simulink model "DR18E_Testpult"  (R2017a)
settings: Solver=ode1  StartTime=0.0  StopTime=Inf  FixedStep=0.001  RelTol=1e-3
PostLoadFcn:
  | , if any(exist('dsrtsu_mdlpostloadfcn', 'file') == [2, 3, 6]), try dsrtsu_mdlpostloadfcn('Execute', bdroot); catch fprintf('Error in PostLoadFcn (dsrtsu_mdlpostloadfcn) for model "%s":\n %s\n', bdroot, lasterr); end, end,
model workspace: external: MAT-File C:\Users\DeltaRacing\Documents\dSPACE\MABX_DR18E\Model\DR18E_MABX_Parameter.mat (data not in the file)
values from neighbouring files (symbols this model uses):
  am = 1/Ts    (= 1)    [DR18E_MABX_Parameter.m]
  bm = K/Ts    (= 0.05)    [DR18E_MABX_Parameter.m]
  cf = 41350    [DR18E_MABX_Parameter.m]
  cr = 41350    [DR18E_MABX_Parameter.m]
  Derating_HV_Battery_Kapa = 1    [DR18E_MABX_Parameter.m]
  Derating_Start_km = 16    [DR18E_MABX_Parameter.m]
  Drive_Mode = 0    [DR18E_MABX_Parameter.m]
  g = 1    [DR18E_MABX_Parameter.m]
  Gas_Modus = 2    [DR18E_MABX_Parameter.m]
  HV_Power_max = 80    [DR18E_MABX_Parameter.m]
  i_Getriebe = 3.3    [DR18E_MABX_Parameter.m]
  i_Lenkgetriebe = 4.32    [DR18E_MABX_Parameter.m]
  K_SET = 1    [DR18E_MABX_Parameter.m]
  Kapazitaet_HV_Battery_kWh = 6.6    [DR18E_MABX_Parameter.m]
  KW_T_Soll = 37    [DR18E_MABX_Parameter.m]
  lf = 1.2    [DR18E_MABX_Parameter.m]
  lr = 1.15    [DR18E_MABX_Parameter.m]
  m = mdriver + mvehicle    (= 310)    [DR18E_MABX_Parameter.m]
  M_max = 150    [DR18E_MABX_Parameter.m]
  Power_Limit_onoff = 0    [DR18E_MABX_Parameter.m]
  Reifenradius = 0.2351    [DR18E_MABX_Parameter.m]
  Strecke_Endu_km = 22    [DR18E_MABX_Parameter.m]
  TC_Decr_Gas = 0.00005    (= 5e-05)    [DR18E_MABX_Parameter.m]
  TC_Derivative = 0.4    [DR18E_MABX_Parameter.m]
  TC_Incr_Gas = 0.005    [DR18E_MABX_Parameter.m]
  TC_On = 0    [DR18E_MABX_Parameter.m]
  TC_Relay_Off = 0.065    [DR18E_MABX_Parameter.m]
  TC_Relay_On = 0.07    [DR18E_MABX_Parameter.m]
  TV_Mode = 2    [DR18E_MABX_Parameter.m]
  TV_On = 0    [DR18E_MABX_Parameter.m]
  TV_Override = 1    [DR18E_MABX_Parameter.m]
  y = 0.8    [DR18E_MABX_Parameter.m]
undefined symbols (not defined in the file or in its folder): D, DiscIntNeverNeededParam, I, K_OL, P
libraries: simulink x288, rtican x100, rtiusbflightreclib x40, rti1401lib_dio_type3 x10, simulink_extras x10, rti1401lib_adc_type4 x8, rti1401lib_II_base x7
(part 25 of 27)

== system DR18E_Testpult/Verarbeitung/Bremse/PlausibilityCheck/PT1 Discrete1 ==
  u : Inport
  K : Inport  Port=2
  T : Inport  Port=3
  Memory : Memory
  Product : Product
  Product1 : Product
  Subsystem : Subsystem
  Sum : Sum  Inputs=|+-
  Sum1 : Sum  Inputs=|++
  y : Outport
  wires:
  T/1 -> Subsystem/1(T)
  Product/1 -> Sum/1
  Sum1/1 -> Memory/1, y/1
  Memory/1 -> Sum/2, Sum1/2
  Product1/1 -> Sum1/1
  Sum/1 -> Product1/2
  u/1 -> Product/2
  Subsystem/1(T*) -> Product1/1
  K/1 -> Product/1

== system DR18E_Testpult/Verarbeitung/DR18E Torque Control/Derating/Derating_Strategie_Reichweite ==
  note: Eingänge Timeout Drehzahlsensor
      | HV Strom
  In1 : Inport
  In2 : Inport  Port=2
  Add : Sum  Inputs=+-
  Add1 : Sum  Inputs=-+
  Add2 : Sum  Inputs=-+
  Compare To Constant : simulink/Logic and Bit Operations/Compare To Constant  relop===  const=3.0  OutDataTypeStr=boolean
  Constant : Constant  Value=Kapazitaet_HV_Battery_kWh
  Constant1 : Constant  Value=Strecke_Endu_km
  Constant2 : Constant  Value=Drive_Mode
  Constant3 : Constant  Value=Derating_HV_Battery_Kapa
  Constant4 : Constant  Value=Derating_Start_km
  Derating_Battery_active : Switch  Criteria=u2 > Threshold
  Divide : Product  Inputs=*/
  Divide1 : Product  Inputs=*/
  Logical Operator : Logic  Inputs=4  AllPortsSameDT=off  OutDataTypeStr=boolean
  Map_Reichweite_Derating_Rev1 : Lookup_n-D  NumberOfTableDimensions=1  BreakpointsForDimension1=[0;1;2;3;4;5;6;7;8;9;10]  Table=[1;0.9;0.8;0.8;0.8;0.8;0.8;0.7;0.7;0.7;0.7]  InternalRulePriority=Speed  RndMeth=Simplest  InputSameDT=on
  Relational Operator : RelationalOperator  OutDataTypeStr=boolean  RndMeth=Simplest
  Safety1 : Constant  Value=0
  Safety_Derateing : Constant
  Saturation : Saturate  UpperLimit=10  LowerLimit=0
  Verbrauch_Wh/km : Subsystem
  kWh->Wh : Gain  Gain=1000
  m->km : Gain  Gain=1/1000
  deltaStrecke_km : Outport
  Derating_RW_aktivate_bin : Outport  Port=2
  wires:
  Add1/1 -> Add2/2  "Reststrecke_km"
  Add/1 -> Divide1/1  "verbleibendeEnergie_Wh"
  kWh->Wh/1 -> Add/1
  Divide1/1 -> Add2/1  "Restreichweite_km"
  In1/1 -> Divide/1, Add/2
  m->km/1 -> Relational Operator/1, Add1/1, Divide/2
  Constant1/1 -> Add1/2
  Constant/1 -> kWh->Wh/1
  In2/1 -> m->km/1
  Add2/1 -> Saturation/1  "deltaStrecke_km"
  Divide/1 -> Verbrauch_Wh/km/1(In1), Divide1/2  "Verbrauch_Wh/km"
  Compare To Constant/1 -> Logical Operator/4  "Drive_Mode_Derating_0_1"
  Logical Operator/1 -> Derating_Battery_active/2, Derating_RW_aktivate_bin/1
  Constant4/1 -> Relational Operator/2
  Relational Operator/1 -> Logical Operator/1  "Start_Derating_0_1"
  Constant3/1 -> Logical Operator/3  "manual_Derating_0_1"
  Safety_Derateing/1 -> Logical Operator/2  "Safety_Derating_0_1"
  Constant2/1 -> Compare To Constant/1
  Safety1/1 -> Derating_Battery_active/3
  Derating_Battery_active/1 -> Map_Reichweite_Derating_Rev1/1
  Map_Reichweite_Derating_Rev1/1 -> deltaStrecke_km/1
  Saturation/1 -> Derating_Battery_active/1

== system DR18E_Testpult/Verarbeitung/DR18E Torque Control/TC RL/Traction Control RL ==
  Gas_0-1 : Inport
  Car.LongSlip : Inport  Port=2
  Add : Sum
  Compare To Constant : simulink/Logic and Bit Operations/Compare To Constant  relop=>  const=TC_Derivative  OutDataTypeStr=uint8  ZeroCross=off
  Data Type Conversion : DataTypeConversion  OutDataTypeStr=boolean
  Delay : Delay  DelayLength=1  InitialCondition=0
  Derivative : Derivative
  Fcn : Fcn  Expr=u >0.05
  Fcn1 : Fcn  Expr=u+TC_Incr_Gas
  Fcn2 : Fcn  Expr=u-TC_Decr_Gas
  Multiport Switch : MultiPortSwitch  DataPortOrder=Zero-based contiguous  DiagnosticForDefault=Warning  zeroidx=on
  Relational Operator : RelationalOperator  Operator=<=  RndMeth=Nearest
  Relay : Relay  OnSwitchValue=TC_Relay_On  OffSwitchValue=TC_Relay_Off
  S-R Flip-Flop : simulink_extras/Flip Flops/S-R Flip-Flop  initial_condition=0
  Saturation : Saturate  UpperLimit=1  LowerLimit=0
  Saturation1 : Saturate  UpperLimit=1  LowerLimit=0
  Switch : Switch  Criteria=u2 > Threshold
  Terminator : Terminator
  E_Gas : Outport
  wires:
  [A] -> Switch/3
  Saturation/1 -> Multiport Switch/4
  Fcn2/1 -> Saturation/1
  Saturation1/1 -> Switch/1
  Fcn1/1 -> Saturation1/1
  Switch/1 -> Multiport Switch/2
  S-R Flip-Flop/1 -> Switch/2
  S-R Flip-Flop/2 -> Terminator/1
  Multiport Switch/1 -> Delay/1, E_Gas/1
  Gas_0-1/1 -> [A], Relational Operator/1
  Add/1 -> Multiport Switch/1
  Compare To Constant/1 -> Add/2
  Derivative/1 -> Compare To Constant/1
  Relay/1 -> Add/1
  Fcn/1 -> Data Type Conversion/1
  Car.LongSlip/1 -> Fcn/1, Derivative/1, Relay/1
  Relational Operator/1 -> S-R Flip-Flop/2
  Data Type Conversion/1 -> S-R Flip-Flop/1
  Delay/1 -> Multiport Switch/3, Fcn2/1, Fcn1/1, Relational Operator/2

== system DR18E_Testpult/Verarbeitung/DR18E Torque Control/TC RR/Traction Control RR ==
  Gas_0-1 : Inport
  Car.LongSlip : Inport  Port=2
  Add : Sum
  Compare To Constant : simulink/Logic and Bit Operations/Compare To Constant  relop=>  const=TC_Derivative  OutDataTypeStr=uint8  ZeroCross=off
  Data Type Conversion : DataTypeConversion  OutDataTypeStr=boolean
  Delay : Delay  DelayLength=1  InitialCondition=0
  Derivative : Derivative
  Fcn : Fcn  Expr=u >0.05
  Fcn1 : Fcn  Expr=u+TC_Incr_Gas
  Fcn2 : Fcn  Expr=u-TC_Decr_Gas
  Multiport Switch : MultiPortSwitch  DataPortOrder=Zero-based contiguous  DiagnosticForDefault=Warning  zeroidx=on
  Relational Operator : RelationalOperator  Operator=<=  RndMeth=Nearest
  Relay : Relay  OnSwitchValue=TC_Relay_On  OffSwitchValue=TC_Relay_Off
  S-R Flip-Flop : simulink_extras/Flip Flops/S-R Flip-Flop  initial_condition=0
  Saturation : Saturate  UpperLimit=1  LowerLimit=0
  Saturation1 : Saturate  UpperLimit=1  LowerLimit=0
  Switch : Switch  Criteria=u2 > Threshold
  Terminator : Terminator
  E_Gas : Outport
  wires:
  [A] -> Switch/3
  Saturation/1 -> Multiport Switch/4
  Fcn2/1 -> Saturation/1
  Saturation1/1 -> Switch/1
  Fcn1/1 -> Saturation1/1
  Relational Operator/1 -> S-R Flip-Flop/2
  Switch/1 -> Multiport Switch/2
  S-R Flip-Flop/1 -> Switch/2
  S-R Flip-Flop/2 -> Terminator/1
  Multiport Switch/1 -> Delay/1, E_Gas/1
  Gas_0-1/1 -> [A], Relational Operator/1
  Add/1 -> Multiport Switch/1
  Compare To Constant/1 -> Add/2
  Derivative/1 -> Compare To Constant/1
  Relay/1 -> Add/1
  Car.LongSlip/1 -> Fcn/1, Derivative/1, Relay/1
  Fcn/1 -> Data Type Conversion/1
  Data Type Conversion/1 -> S-R Flip-Flop/1
  Delay/1 -> Fcn1/1, Multiport Switch/3, Fcn2/1, Relational Operator/2

== system DR18E_Testpult/Verarbeitung/DR18E Torque Control/TV RL/MRAC_PT1_Lyapunov ==
  note: Vorteil:
      |
      | - Stabilität ist nachgewiesen
      |
      | Nachteil:
      |
      | - kann evtl. die Adaption nicht so schnell finden
  note: em
  note: Xm(s)
  note: X(s)
  note: Y(s)
  note: W(s)
  note: P2*X(s)
  note: P1*W(s)²
  YawRate REF (rad/s) : Inport
  Car.YawRate : Inport  Port=2
  ModelReference : TransferFcn  Numerator=[bm]  Denominator=[1 am]
  Product{,1..3} (4 alike) : Product
  Sum : Sum  Inputs=-+
  Sum1 : Sum  Inputs=|+-
  em*GM : TransferFcn  Numerator=[-y]  Denominator=[1 0]
  em*GM*X² : TransferFcn  Numerator=[y]  Denominator=[1 0]
  Delta M (Nm) : Outport
  wires:
  Sum1/1 -> Delta M (Nm)/1
  ModelReference/1 -> Sum/1
  Car.YawRate/1 -> Product2/2, Product1/1, Sum/2  "YawRate Feedback (rad/s)"
  Product1/1 -> em*GM*X²/1
  Product/1 -> Sum1/1
  YawRate REF (rad/s)/1 -> Product3/1, Product/1, ModelReference/1
  Sum/1 -> Product3/2, Product1/2
  em*GM/1 -> Product/2
  em*GM*X²/1 -> Product2/1
  Product2/1 -> Sum1/2
  Product3/1 -> em*GM/1

== system DR18E_Testpult/Verarbeitung/DR18E Torque Control/TV RL/MRAC_PT1_MIT_DIFF ==
  note: Vorteil:
      |
      | - kann die Adaption schneller finden
      | - schnelle Änderungen können schnell adaptiert werden, dank eines Differntialanteils im Regler
      |
      | Nachteil:
      |
      | - unter Störungen bei schnellen Schwankungen kann der Regler instabil werden
      | - Stabilität ist allgemein nicht nachgewiesen
  note: Y(s)
  note: W(s)
  note: P1*W(s)²
  YawRate REF (rad/s) : Inport
  Car.YawRate : Inport  Port=2
  Derivative : Derivative
  Gain : Gain  Gain=-1
  Gain1 : Gain  Gain=y
  ModelReference : TransferFcn  Numerator=[bm]  Denominator=[1 am]
  ModelReference1 : TransferFcn  Numerator=[bm]  Denominator=[1 am]
  ModelReference2 : TransferFcn  Denominator=[1 0]
  ModelReference3 : TransferFcn  Numerator=[bm]  Denominator=[1 am]
  ModelReference4 : TransferFcn  Denominator=[1 0]
  Product{,1..4} (5 alike) : Product
  Sum1 : Sum  Inputs=|+-
  Sum2 : Sum  Inputs=|-+
  Sum3 : Sum  Inputs=|+-
  Delta M (Nm) : Outport
  wires:
  Car.YawRate/1 -> Derivative/1, Product4/1, Sum2/2, Product3/2  "YawRate Feedback (rad/s)"
  ModelReference/1 -> Sum2/1
  Product/1 -> Sum1/1
  YawRate REF (rad/s)/1 -> Product/1, Gain/1, ModelReference/1
  Gain/1 -> Product2/1
  Sum2/1 -> Gain1/1
  Gain1/1 -> Product3/1, Product2/2
  ModelReference2/1 -> Product4/2
  Product4/1 -> Sum1/2
  Derivative/1 -> Product1/1
  ModelReference1/1 -> ModelReference2/1, Product1/2
  Sum1/1 -> Sum3/1
  Sum3/1 -> Delta M (Nm)/1
  Product1/1 -> Sum3/2
  ModelReference3/1 -> ModelReference4/1
  ModelReference4/1 -> Product/2
  Product2/1 -> ModelReference3/1
  Product3/1 -> ModelReference1/1

== system DR18E_Testpult/Verarbeitung/DR18E Torque Control/TV RL/MRAC_PT1_MIT_NORM ==
  note: Vorteil:
      |
      | - weniger störanfällig
      | - einigermaßen schnelle Adaption
      |
      | Nachteil:
      |
      | - Stabilität nicht nachgewiesen
      | - Schnelle Änderungen werden nicht wahrgenommen
  note: Y(s)
  note: W(s)
  note: P1*W(s)²
  YawRate REF (rad/s) : Inport
  Car.YawRate : Inport  Port=2
  Gain : Gain  Gain=-1
  Gain1 : Gain  Gain=y
  ModelReference : TransferFcn  Numerator=[bm]  Denominator=[1 am]
  ModelReference1 : TransferFcn  Numerator=[bm]  Denominator=[1 am]
  ModelReference2 : TransferFcn  Denominator=[1 0]
  ModelReference3 : TransferFcn  Numerator=[bm]  Denominator=[1 am]
  ModelReference4 : TransferFcn  Denominator=[1 0]
  Product{,2..4} (4 alike) : Product
  Sum1 : Sum  Inputs=|+-
  Sum2 : Sum  Inputs=|-+
  Delta M (Nm) : Outport
  wires:
  Car.YawRate/1 -> Product4/1, Sum2/2, Product3/2  "YawRate Feedback (rad/s)"
  ModelReference/1 -> Sum2/1
  Product/1 -> Sum1/1
  YawRate REF (rad/s)/1 -> Product/1, Gain/1, ModelReference/1
  Gain/1 -> Product2/1
  Sum2/1 -> Gain1/1
  Gain1/1 -> Product3/1, Product2/2
  ModelReference2/1 -> Product4/2
  Product4/1 -> Sum1/2
  ModelReference1/1 -> ModelReference2/1
  Sum1/1 -> Delta M (Nm)/1
  ModelReference3/1 -> ModelReference4/1
  ModelReference4/1 -> Product/2
  Product2/1 -> ModelReference3/1
  Product3/1 -> ModelReference1/1

== system DR18E_Testpult/Verarbeitung/DR18E Torque Control/TV RL/TV DR17E ==
  note: Change the Torque Vectoring here
  vx_ms : Inport
  Radeinschlagwinkel_deg : Inport  Port=2
  psipunkt_ist_deg_s : Inport  Port=3
  Drehmomentverteilung links/rechts : Subsystem
  Ermittlung Sollgierrate : Subsystem
  FlightRecorder4 : Subsystem
  Saturation : Saturate  UpperLimit=M_max  LowerLimit=-M_max
  Saturation1 : Saturate  UpperLimit=0  LowerLimit=-M_max
  Vorsteuerung+PID : Subsystem
  Delta M (Nm) : Outport
  wires:
  vx_ms/1 -> Ermittlung Sollgierrate/1(vx-ms)
  Radeinschlagwinkel_deg/1 -> Ermittlung Sollgierrate/2(Radeinschlagwinkel-deg)
  Ermittlung Sollgierrate/1(Psipunkt-Soll-deg-s) -> FlightRecorder4/1(In1), Vorsteuerung+PID/1(PsiPunktSoll)
  psipunkt_ist_deg_s/1 -> Vorsteuerung+PID/2(PsiPunktIst)
  Saturation/1 -> Drehmomentverteilung links/rechts/1(DeltaM_in)
  Drehmomentverteilung links/rechts/1(deltaM_Out) -> Saturation1/1
  Vorsteuerung+PID/1(DeltaM) -> Saturation/1
  Saturation1/1 -> Delta M (Nm)/1

== system DR18E_Testpult/Verarbeitung/DR18E Torque Control/TV RL/TV IPG ==
  In2 : Inport
  In3 : Inport  Port=2
  In4 : Inport  Port=3
  Abs : Abs
  Abs2 : Abs
  Constant : Constant
  Divide : Product  Inputs=*/
  Gain : Gain  Gain=-1
  Gain1 : Gain  Gain=M_max
  Gravity : Gain  Gain=9.81
  Lookup Table : Lookup  InputValues=[0,0.1,0.2,0.3,0.4,0.5,0.6,0.7,0.8,1,2,3,4]  Table=[0,0,0.05,0.1,0.2,0.3,0.4,0.5,0.6,0.7,1,1,1]
  Override : Gain  Gain=TV_Override
  Product : Product  RndMeth=Zero
  Subtract : Sum  Inputs=+-
  Switch : Switch  Criteria=u2 > Threshold
  muRoad : Constant  Value=1.6
  Out1 : Outport
  wires:
  Gain/1 -> Lookup Table/1
  Abs2/1 -> Subtract/2
  Divide/1 -> Subtract/1
  Gravity/1 -> Override/1
  Gain1/1 -> Out1/1  "Torque_AC_OLD_RL"
  Product/1 -> Gain1/1
  In4/1 -> Gain/1
  Override/1 -> Divide/1
  Switch/1 -> Abs/1
  In2/1 -> Switch/1, Switch/2  "v_kmh"
  muRoad/1 -> Gravity/1
  Abs/1 -> Divide/2
  Constant/1 -> Switch/3
  Subtract/1 -> Product/1
  Lookup Table/1 -> Product/2
  In3/1 -> Abs2/1

== system DR18E_Testpult/Verarbeitung/DR18E Torque Control/TV RL/YawRate SET_NEW  ==
  Radeinschlagwinkel_rad : Inport
  v_ms : Inport  Port=2
  Divide : Product  Inputs=*/
  Divide1 : Product  Inputs=*/
  Divide2 : Product  Inputs=*/
  Eigenlenkgradient : Constant  Value=m*(cr*lr-cf*lf)/(cr*cf*(lr+lf))
  Faktor : Constant
  Product : Product
  Product1 : Product
  Radstand : Constant  Value=lr+lf
  Sum : Sum  Inputs=|++
  sqr2 : Math  Operator=square  SaturateOnIntegerOverflow=on
  YawRate REF (rad/s) : Outport
  wires:
  Divide/1 -> YawRate REF (rad/s)/1
  Product/1 -> Divide/1
  Product1/1 -> Divide/2
  Sum/1 -> Product1/1
  Faktor/1 -> Sum/2
  Divide1/1 -> Sum/1
  Divide2/1 -> Divide1/2
  Eigenlenkgradient/1 -> Divide2/2
  sqr2/1 -> Divide1/1
  Radstand/1 -> Product1/2, Divide2/1
  Radeinschlagwinkel_rad/1 -> Product/1  "Radeinschlagwinkel_rad"
  v_ms/1 -> Product/2, sqr2/1  "v_ms"

== system DR18E_Testpult/Verarbeitung/DR18E Torque Control/TV RR/MRAC_PT1_Lyapunov ==
  note: Vorteil:
      |
      | - Stabilität ist nachgewiesen
      |
      | Nachteil:
      |
      | - kann evtl. die Adaption nicht so schnell finden
  note: em
  note: Xm(s)
  note: X(s)
  note: Y(s)
  note: W(s)
  note: P2*X(s)
  note: P1*W(s)²
  YawRate REF (rad/s) : Inport
  Car.YawRate : Inport  Port=2
  ModelReference : TransferFcn  Numerator=[bm]  Denominator=[1 am]
  Product{,1..3} (4 alike) : Product
  Sum : Sum  Inputs=-+
  Sum1 : Sum  Inputs=|+-
  em*GM : TransferFcn  Numerator=[-y]  Denominator=[1 0]
  em*GM*X² : TransferFcn  Numerator=[y]  Denominator=[1 0]
  Delta M (Nm) : Outport
  wires:
  Sum1/1 -> Delta M (Nm)/1
  ModelReference/1 -> Sum/1
  Car.YawRate/1 -> Product2/2, Product1/1, Sum/2  "YawRate Feedback (rad/s)"
  Product1/1 -> em*GM*X²/1
  Product/1 -> Sum1/1
  YawRate REF (rad/s)/1 -> Product3/1, Product/1, ModelReference/1
  Sum/1 -> Product3/2, Product1/2
  em*GM/1 -> Product/2
  em*GM*X²/1 -> Product2/1
  Product2/1 -> Sum1/2
  Product3/1 -> em*GM/1

== system DR18E_Testpult/Verarbeitung/DR18E Torque Control/TV RR/MRAC_PT1_MIT_DIFF ==
  note: Vorteil:
      |
      | - kann die Adaption schneller finden
      | - schnelle Änderungen können schnell adaptiert werden, dank eines Differntialanteils im Regler
      |
      | Nachteil:
      |
      | - unter Störungen bei schnellen Schwankungen kann der Regler instabil werden
      | - Stabilität ist allgemein nicht nachgewiesen
  note: Y(s)
  note: W(s)
  note: P1*W(s)²
  YawRate REF (rad/s) : Inport
  Car.YawRate : Inport  Port=2
  Derivative : Derivative
  Gain : Gain  Gain=-1
  Gain1 : Gain  Gain=y
  ModelReference : TransferFcn  Numerator=[bm]  Denominator=[1 am]
  ModelReference1 : TransferFcn  Numerator=[bm]  Denominator=[1 am]
  ModelReference2 : TransferFcn  Denominator=[1 0]
  ModelReference3 : TransferFcn  Numerator=[bm]  Denominator=[1 am]
  ModelReference4 : TransferFcn  Denominator=[1 0]
  Product{,1..4} (5 alike) : Product
  Sum1 : Sum  Inputs=|+-
  Sum2 : Sum  Inputs=|-+
  Sum3 : Sum  Inputs=|+-
  Delta M (Nm) : Outport
  wires:
  Car.YawRate/1 -> Derivative/1, Product4/1, Sum2/2, Product3/2  "YawRate Feedback (rad/s)"
  ModelReference/1 -> Sum2/1
  Product/1 -> Sum1/1
  YawRate REF (rad/s)/1 -> Product/1, Gain/1, ModelReference/1
  Gain/1 -> Product2/1
  Sum2/1 -> Gain1/1
  Gain1/1 -> Product3/1, Product2/2
  ModelReference2/1 -> Product4/2
  Product4/1 -> Sum1/2
  Derivative/1 -> Product1/1
  ModelReference1/1 -> ModelReference2/1, Product1/2
  Sum1/1 -> Sum3/1
  Sum3/1 -> Delta M (Nm)/1
  Product1/1 -> Sum3/2
  ModelReference3/1 -> ModelReference4/1
  ModelReference4/1 -> Product/2
  Product2/1 -> ModelReference3/1
  Product3/1 -> ModelReference1/1

== system DR18E_Testpult/Verarbeitung/DR18E Torque Control/TV RR/MRAC_PT1_MIT_NORM ==
  note: Vorteil:
      |
      | - weniger störanfällig
      | - einigermaßen schnelle Adaption
      |
      | Nachteil:
      |
      | - Stabilität nicht nachgewiesen
      | - Schnelle Änderungen werden nicht wahrgenommen
  note: Y(s)
  note: W(s)
  note: P1*W(s)²
  YawRate REF (rad/s) : Inport
  Car.YawRate : Inport  Port=2
  Gain : Gain  Gain=-1
  Gain1 : Gain  Gain=y
  ModelReference : TransferFcn  Numerator=[bm]  Denominator=[1 am]
  ModelReference1 : TransferFcn  Numerator=[bm]  Denominator=[1 am]
  ModelReference2 : TransferFcn  Denominator=[1 0]
  ModelReference3 : TransferFcn  Numerator=[bm]  Denominator=[1 am]
  ModelReference4 : TransferFcn  Denominator=[1 0]
  Product{,2..4} (4 alike) : Product
  Sum1 : Sum  Inputs=|+-
  Sum2 : Sum  Inputs=|-+
  Delta M (Nm) : Outport
  wires:
  Car.YawRate/1 -> Product4/1, Sum2/2, Product3/2  "YawRate Feedback (rad/s)"
  ModelReference/1 -> Sum2/1
  Product/1 -> Sum1/1
  YawRate REF (rad/s)/1 -> Product/1, Gain/1, ModelReference/1
  Gain/1 -> Product2/1
  Sum2/1 -> Gain1/1
  Gain1/1 -> Product3/1, Product2/2
  ModelReference2/1 -> Product4/2
  Product4/1 -> Sum1/2
  ModelReference1/1 -> ModelReference2/1
  Sum1/1 -> Delta M (Nm)/1
  ModelReference3/1 -> ModelReference4/1
  ModelReference4/1 -> Product/2
  Product2/1 -> ModelReference3/1
  Product3/1 -> ModelReference1/1

== system DR18E_Testpult/Verarbeitung/DR18E Torque Control/TV RR/TV DR17E ==
  note: Change the Torque Vectoring here
  vx_ms : Inport
  Radeinschlagwinkel_deg : Inport  Port=2
  psipunkt_ist_deg_s : Inport  Port=3
  Drehmomentverteilung links/rechts : Subsystem
  Ermittlung Sollgierrate : Subsystem
  FlightRecorder4 : Subsystem
  Saturation : Saturate  UpperLimit=M_max  LowerLimit=-M_max
  Saturation1 : Saturate  UpperLimit=0  LowerLimit=-M_max
  Vorsteuerung+PID : Subsystem
  Delta M (Nm) : Outport
  wires:
  vx_ms/1 -> Ermittlung Sollgierrate/1(vx-ms)
  Radeinschlagwinkel_deg/1 -> Ermittlung Sollgierrate/2(Radeinschlagwinkel-deg)
  Ermittlung Sollgierrate/1(Psipunkt-Soll-deg-s) -> FlightRecorder4/1(In1), Vorsteuerung+PID/1(PsiPunktSoll)
  psipunkt_ist_deg_s/1 -> Vorsteuerung+PID/2(PsiPunktIst)
  Saturation/1 -> Drehmomentverteilung links/rechts/1(DeltaM_in)
  Drehmomentverteilung links/rechts/1(deltaM_Out) -> Saturation1/1
  Vorsteuerung+PID/1(DeltaM) -> Saturation/1
  Saturation1/1 -> Delta M (Nm)/1

== system DR18E_Testpult/Verarbeitung/DR18E Torque Control/TV RR/TV IPG ==
  In2 : Inport
  In3 : Inport  Port=2
  In4 : Inport  Port=3
  Abs : Abs
  Abs2 : Abs
  Constant : Constant
  Divide : Product  Inputs=*/
  Gain : Gain  Gain=-1
  Gain1 : Gain  Gain=M_max
  Gravity : Gain  Gain=9.81
  Lookup Table : Lookup  InputValues=[0,0.1,0.2,0.3,0.4,0.5,0.6,0.7,0.8,1,2,3,4]  Table=[0,0,0.05,0.1,0.2,0.3,0.4,0.5,0.6,0.7,1,1,1]
  Override : Gain  Gain=TV_Override
  Product : Product  RndMeth=Zero
  Subtract : Sum  Inputs=+-
  Switch : Switch  Criteria=u2 > Threshold
  muRoad : Constant  Value=1.6
  Out1 : Outport
  wires:
  Gain/1 -> Lookup Table/1
  Abs2/1 -> Subtract/2
  Divide/1 -> Subtract/1
  Gravity/1 -> Override/1
  Gain1/1 -> Out1/1  "Torque_AC_OLD_RL"
  Product/1 -> Gain1/1
  In4/1 -> Gain/1
  Override/1 -> Divide/1
  Switch/1 -> Abs/1
  In2/1 -> Switch/1, Switch/2  "v_kmh"
  muRoad/1 -> Gravity/1
  Abs/1 -> Divide/2
  Constant/1 -> Switch/3
  Subtract/1 -> Product/1
  Lookup Table/1 -> Product/2
  In3/1 -> Abs2/1

== system DR18E_Testpult/Verarbeitung/DR18E Torque Control/TV RR/YawRate SET_NEW  ==
  Radeinschlagwinkel_rad : Inport
  v_ms : Inport  Port=2
  Divide : Product  Inputs=*/
  Divide1 : Product  Inputs=*/
  Divide2 : Product  Inputs=*/
  Eigenlenkgradient : Constant  Value=m*(cr*lr-cf*lf)/(cr*cf*(lr+lf))
  Faktor : Constant
  Product : Product
  Product1 : Product
  Radstand : Constant  Value=lr+lf
  Sum : Sum  Inputs=|++
  sqr2 : Math  Operator=square  SaturateOnIntegerOverflow=on
  YawRate REF (rad/s) : Outport
  wires:
  Divide/1 -> YawRate REF (rad/s)/1
  Product/1 -> Divide/1
  Product1/1 -> Divide/2
  Sum/1 -> Product1/1
  Faktor/1 -> Sum/2
  Divide1/1 -> Sum/1
  Divide2/1 -> Divide1/2
  Eigenlenkgradient/1 -> Divide2/2
  sqr2/1 -> Divide1/1
  Radstand/1 -> Product1/2, Divide2/1
  Radeinschlagwinkel_rad/1 -> Product/1  "Radeinschlagwinkel_rad"
  v_ms/1 -> Product/2, sqr2/1  "v_ms"

== system DR18E_Testpult/Verarbeitung/DR18E Torque Control/Torque Filter/PT1 Discrete1 ==
  u : Inport
  K : Inport  Port=2
  T : Inport  Port=3
  Reset : Inport  Port=4
  Data Type Conversion : DataTypeConversion  OutDataTypeStr=double
  Logical Operator : Logic  Operator=NOT  AllPortsSameDT=off  OutDataTypeStr=boolean
  Memory : Memory
  Product : Product
  Product1 : Product
  Product2 : Product
  Subsystem : Subsystem
  Sum : Sum  Inputs=|+-
  Sum1 : Sum  Inputs=|++
  y : Outport
  wires:
  K/1 -> Product/1
  Subsystem/1(T*) -> Product1/1
  u/1 -> Product/2
  Sum/1 -> Product1/2
  Product1/1 -> Sum1/1
  Memory/1 -> Sum1/2, Sum/2
  Product/1 -> Sum/1
  T/1 -> Subsystem/1(T)
  Reset/1 -> Logical Operator/1
  Logical Operator/1 -> Data Type Conversion/1
  Sum1/1 -> Product2/2
  Data Type Conversion/1 -> Product2/1
  Product2/1 -> Memory/1, y/1

== system DR18E_Testpult/Verarbeitung/DR18E Torque Control/Torque Filter/PT1 Discrete3 ==
  u : Inport
  K : Inport  Port=2
  T : Inport  Port=3
  Reset : Inport  Port=4
  Data Type Conversion : DataTypeConversion  OutDataTypeStr=double
  Logical Operator : Logic  Operator=NOT  AllPortsSameDT=off  OutDataTypeStr=boolean
  Memory : Memory
  Product : Product
  Product1 : Product
  Product2 : Product
  Subsystem : Subsystem
  Sum : Sum  Inputs=|+-
  Sum1 : Sum  Inputs=|++
  y : Outport
  wires:
  K/1 -> Product/1
  Subsystem/1(T*) -> Product1/1
  u/1 -> Product/2
  Sum/1 -> Product1/2
  Product1/1 -> Sum1/1
  Memory/1 -> Sum1/2, Sum/2
  Product/1 -> Sum/1
  T/1 -> Subsystem/1(T)
  Reset/1 -> Logical Operator/1
  Logical Operator/1 -> Data Type Conversion/1
  Sum1/1 -> Product2/2
  Data Type Conversion/1 -> Product2/1
  Product2/1 -> Memory/1, y/1

== system DR18E_Testpult/Verarbeitung/Gaspedal Check/PlausibilityCheck/PT1 Discrete ==
  u : Inport
  K : Inport  Port=2
  T : Inport  Port=3
  Memory : Memory
  Product : Product
  Product1 : Product
  Subsystem : Subsystem
  Sum : Sum  Inputs=|+-
  Sum1 : Sum  Inputs=|++
  y : Outport
  wires:
  K/1 -> Product/1
  Subsystem/1(T*) -> Product1/1
  u/1 -> Product/2
  Sum/1 -> Product1/2
  Product1/1 -> Sum1/1
  Memory/1 -> Sum1/2, Sum/2
  Sum1/1 -> y/1, Memory/1
  Product/1 -> Sum/1
  T/1 -> Subsystem/1(T)

== system DR18E_Testpult/Verarbeitung/Gaspedal Check/PlausibilityCheck/PT1 Discrete1 ==
  u : Inport
  K : Inport  Port=2
  T : Inport  Port=3
  Memory : Memory
  Product : Product
  Product1 : Product
  Subsystem : Subsystem
  Sum : Sum  Inputs=|+-
  Sum1 : Sum  Inputs=|++
  y : Outport
  wires:
  K/1 -> Product/1
  Subsystem/1(T*) -> Product1/1
  u/1 -> Product/2
  Sum/1 -> Product1/2
  Product1/1 -> Sum1/1
  Memory/1 -> Sum1/2, Sum/2
  Sum1/1 -> y/1, Memory/1
  Product/1 -> Sum/1
  T/1 -> Subsystem/1(T)

== system DR18E_Testpult/Verarbeitung/Precalculations/kilometer tracking/FlightRecorder1 ==
  In1 : Inport
  Data Type Conversion : DataTypeConversion
  Gain : Gain
  USB_FLIGHT_REC_BL1 : rtiusbflightreclib/USB_FLIGHT_REC_BL1  VarName=tages_s_m  DataType=Single  SampleTime=0.5  TLCFileName=rtiusbflightrecwrite  Reserved1=[]  Reserved2=[]  Reserved3=[]  Reserved4=[]  DSProperties=struct('RTI',struct('Version',uint32(3),'BlockType',struct('isSLSource',uint8(0),'isSLSink',uint8(1),'isHWSource',uint8(0),'isHWSink',uint8(0),'isSetup',uint8(0),'isInline',uint8(1),'isNonInline',uint8(0),'isInterrupt',uint8(0),'isChannelwise',uint8(0)),'IOBoardType',{{'DSUSB','FLIGHTREC'}},'UnitType','FLIGHTREC','Identifier','WRITE','DialogType','SL','BlockSet','RTIUSBFLIGHTREC','SlaveProcessor','NONE'))  RTIBlockInterface=struct('InputPortsActive',1,'InputPortsWidth',int32(1),'InputPortsDataType',{{'SS_SINGLE'}},'BlockDisplay',{{['Write to\nUSB Flight Recorder'],'center'}},'IconTransparency','off','InitLevel',3,'BlockName',struct('Token',{{'USB_FLIGHT_REC_BL1'}}),'MaskDescription',['Write input to the Flight Recorder. Recorded data can be referenced by the specified variable.'],'SampleTime',{{2^-1}})  RTIBlockParameters=struct('VarName',{{'tages_s_m','OFF',[]}},'DataType',{{'Single','OFF',[]}},'SampleTime',{{2^-1,'OFF',[]}},'TLCFileName',{{'rtiusbflightrecwrite','OFF',[]}})  RTISFcnParameters=struct('VarName','char','DataType','char','SampleTime','double','TLCFileName','char')  RTIBlockParaDefault=struct('VarName','Var1','DataType','Single','SampleTime',-1,'TLCFileName','rtiusbflightrecwrite')
      settings: SourceProductName=dSPACE RTI USB Flight Rec Blockset
  wires:
  Data Type Conversion/1 -> USB_FLIGHT_REC_BL1/1
  In1/1 -> Gain/1
  Gain/1 -> Data Type Conversion/1

== system DR18E_Testpult/Verarbeitung/Temperaturregelung1/PT1 Discrete/Subsystem ==
  T : Inport
  Constant : Constant
  Constant2 : Constant
  Divide : Product  Inputs=*/
  Divide1 : Product  Inputs=*/
  Sum : Sum  Inputs=|++
  Weighted Sample Time : SampleTimeMath  TsampMathOp=Ts Only
  T* : Outport
  wires:
  Divide1/1 -> Sum/1
  Constant2/1 -> Sum/2
  T/1 -> Divide1/1
  Sum/1 -> Divide/2
  Constant/1 -> Divide/1
  Weighted Sample Time/1 -> Divide1/2
  Divide/1 -> T*/1

== system DR18E_Testpult/Verarbeitung/Temperaturregelung1/PT1 Discrete1/Subsystem ==
  T : Inport
  Constant : Constant
  Constant2 : Constant
  Divide : Product  Inputs=*/
  Divide1 : Product  Inputs=*/
  Sum : Sum  Inputs=|++
  Weighted Sample Time : SampleTimeMath  TsampMathOp=Ts Only
  T* : Outport
  wires:
  Divide1/1 -> Sum/1
  Constant2/1 -> Sum/2
  T/1 -> Divide1/1
  Sum/1 -> Divide/2
  Constant/1 -> Divide/1
  Weighted Sample Time/1 -> Divide1/2
  Divide/1 -> T*/1

== system DR18E_Testpult/Eingabe Fahrzeug/BMS/STK1-5_Temp /RX Timeout Detection1/Subsystem ==
  TXStatus : Inport
  Timeout : Inport  Port=2
  Constant : Constant
  Constant1 : Constant  Value=0
  Constant2 : Constant
  Constant3 : Constant  Value=0
  Delay : Delay  DelayLength=1  InitialCondition=0
  Relational Operator : RelationalOperator  Operator=>  OutDataTypeStr=boolean  RndMeth=Nearest
  Sum : Sum  Inputs=|++
  Switch : Switch  Criteria=u2 > Threshold
  Switch1 : Switch  Criteria=u2 > Threshold
  Rampe : Outport
  RX Timeout Error : Outport  Port=2
  wires:
  TXStatus/1 -> Switch/2
  Delay/1 -> Sum/2
  Constant/1 -> Sum/1
  Sum/1 -> Switch/3
  Switch/1 -> Delay/1, Relational Operator/1, Rampe/1
  Constant1/1 -> Switch/1
  Constant2/1 -> Switch1/1
  Constant3/1 -> Switch1/3
  Switch1/1 -> RX Timeout Error/1
  Relational Operator/1 -> Switch1/2
  Timeout/1 -> Relational Operator/2

== system DR18E_Testpult/Eingabe Fahrzeug/BMS/STK1-5_Temp /RX Timeout Detection10/Subsystem ==
  TXStatus : Inport
  Timeout : Inport  Port=2
  Constant : Constant
  Constant1 : Constant  Value=0
  Constant2 : Constant
  Constant3 : Constant  Value=0
  Delay : Delay  DelayLength=1  InitialCondition=0
  Relational Operator : RelationalOperator  Operator=>  OutDataTypeStr=boolean  RndMeth=Nearest
  Sum : Sum  Inputs=|++
  Switch : Switch  Criteria=u2 > Threshold
  Switch1 : Switch  Criteria=u2 > Threshold
  Rampe : Outport
  RX Timeout Error : Outport  Port=2
  wires:
  TXStatus/1 -> Switch/2
  Delay/1 -> Sum/2
  Constant/1 -> Sum/1
  Sum/1 -> Switch/3
  Switch/1 -> Delay/1, Relational Operator/1, Rampe/1
  Constant1/1 -> Switch/1
  Constant2/1 -> Switch1/1
  Constant3/1 -> Switch1/3
  Switch1/1 -> RX Timeout Error/1
  Relational Operator/1 -> Switch1/2
  Timeout/1 -> Relational Operator/2

== system DR18E_Testpult/Eingabe Fahrzeug/BMS/STK1-5_Temp /RX Timeout Detection2/Subsystem ==
  TXStatus : Inport
  Timeout : Inport  Port=2
  Constant : Constant
  Constant1 : Constant  Value=0
  Constant2 : Constant
  Constant3 : Constant  Value=0
  Delay : Delay  DelayLength=1  InitialCondition=0
  Relational Operator : RelationalOperator  Operator=>  OutDataTypeStr=boolean  RndMeth=Nearest
  Sum : Sum  Inputs=|++
  Switch : Switch  Criteria=u2 > Threshold
  Switch1 : Switch  Criteria=u2 > Threshold
  Rampe : Outport
  RX Timeout Error : Outport  Port=2
  wires:
  TXStatus/1 -> Switch/2
  Delay/1 -> Sum/2
  Constant/1 -> Sum/1
  Sum/1 -> Switch/3
  Switch/1 -> Delay/1, Relational Operator/1, Rampe/1
  Constant1/1 -> Switch/1
  Constant2/1 -> Switch1/1
  Constant3/1 -> Switch1/3
  Switch1/1 -> RX Timeout Error/1
  Relational Operator/1 -> Switch1/2
  Timeout/1 -> Relational Operator/2

== system DR18E_Testpult/Eingabe Fahrzeug/BMS/STK1-5_Temp /RX Timeout Detection3/Subsystem ==
  TXStatus : Inport
  Timeout : Inport  Port=2
  Constant : Constant
  Constant1 : Constant  Value=0
  Constant2 : Constant
  Constant3 : Constant  Value=0
  Delay : Delay  DelayLength=1  InitialCondition=0
  Relational Operator : RelationalOperator  Operator=>  OutDataTypeStr=boolean  RndMeth=Nearest
  Sum : Sum  Inputs=|++
  Switch : Switch  Criteria=u2 > Threshold
  Switch1 : Switch  Criteria=u2 > Threshold
  Rampe : Outport
  RX Timeout Error : Outport  Port=2
  wires:
  TXStatus/1 -> Switch/2
  Delay/1 -> Sum/2
  Constant/1 -> Sum/1
  Sum/1 -> Switch/3
  Switch/1 -> Delay/1, Relational Operator/1, Rampe/1
  Constant1/1 -> Switch/1
  Constant2/1 -> Switch1/1
  Constant3/1 -> Switch1/3
  Switch1/1 -> RX Timeout Error/1
  Relational Operator/1 -> Switch1/2
  Timeout/1 -> Relational Operator/2

== system DR18E_Testpult/Eingabe Fahrzeug/BMS/STK1-5_Temp /RX Timeout Detection4/Subsystem ==
  TXStatus : Inport
  Timeout : Inport  Port=2
  Constant : Constant
  Constant1 : Constant  Value=0
  Constant2 : Constant
  Constant3 : Constant  Value=0
  Delay : Delay  DelayLength=1  InitialCondition=0
  Relational Operator : RelationalOperator  Operator=>  OutDataTypeStr=boolean  RndMeth=Nearest
  Sum : Sum  Inputs=|++
  Switch : Switch  Criteria=u2 > Threshold
  Switch1 : Switch  Criteria=u2 > Threshold
  Rampe : Outport
  RX Timeout Error : Outport  Port=2
  wires:
  TXStatus/1 -> Switch/2
  Delay/1 -> Sum/2
  Constant/1 -> Sum/1
  Sum/1 -> Switch/3
  Switch/1 -> Delay/1, Relational Operator/1, Rampe/1
  Constant1/1 -> Switch/1
  Constant2/1 -> Switch1/1
  Constant3/1 -> Switch1/3
  Switch1/1 -> RX Timeout Error/1
  Relational Operator/1 -> Switch1/2
  Timeout/1 -> Relational Operator/2

== system DR18E_Testpult/Eingabe Fahrzeug/BMS/STK1-5_Temp /RX Timeout Detection5/Subsystem ==
  TXStatus : Inport
  Timeout : Inport  Port=2
  Constant : Constant
  Constant1 : Constant  Value=0
  Constant2 : Constant
  Constant3 : Constant  Value=0
  Delay : Delay  DelayLength=1  InitialCondition=0
  Relational Operator : RelationalOperator  Operator=>  OutDataTypeStr=boolean  RndMeth=Nearest
  Sum : Sum  Inputs=|++
  Switch : Switch  Criteria=u2 > Threshold
  Switch1 : Switch  Criteria=u2 > Threshold
  Rampe : Outport
  RX Timeout Error : Outport  Port=2
  wires:
  TXStatus/1 -> Switch/2
  Delay/1 -> Sum/2
  Constant/1 -> Sum/1
  Sum/1 -> Switch/3
  Switch/1 -> Delay/1, Relational Operator/1, Rampe/1
  Constant1/1 -> Switch/1
  Constant2/1 -> Switch1/1
  Constant3/1 -> Switch1/3
  Switch1/1 -> RX Timeout Error/1
  Relational Operator/1 -> Switch1/2
  Timeout/1 -> Relational Operator/2

== system DR18E_Testpult/Eingabe Fahrzeug/BMS/STK1-5_Temp /RX Timeout Detection6/Subsystem ==
  TXStatus : Inport
  Timeout : Inport  Port=2
  Constant : Constant
  Constant1 : Constant  Value=0
  Constant2 : Constant
  Constant3 : Constant  Value=0
  Delay : Delay  DelayLength=1  InitialCondition=0
  Relational Operator : RelationalOperator  Operator=>  OutDataTypeStr=boolean  RndMeth=Nearest
  Sum : Sum  Inputs=|++
  Switch : Switch  Criteria=u2 > Threshold
  Switch1 : Switch  Criteria=u2 > Threshold
  Rampe : Outport
  RX Timeout Error : Outport  Port=2
  wires:
  TXStatus/1 -> Switch/2
  Delay/1 -> Sum/2
  Constant/1 -> Sum/1
  Sum/1 -> Switch/3
  Switch/1 -> Delay/1, Relational Operator/1, Rampe/1
  Constant1/1 -> Switch/1
  Constant2/1 -> Switch1/1
  Constant3/1 -> Switch1/3
  Switch1/1 -> RX Timeout Error/1
  Relational Operator/1 -> Switch1/2
  Timeout/1 -> Relational Operator/2

== system DR18E_Testpult/Eingabe Fahrzeug/BMS/STK1-5_Temp /RX Timeout Detection7/Subsystem ==
  TXStatus : Inport
  Timeout : Inport  Port=2
  Constant : Constant
  Constant1 : Constant  Value=0
  Constant2 : Constant
  Constant3 : Constant  Value=0
  Delay : Delay  DelayLength=1  InitialCondition=0
  Relational Operator : RelationalOperator  Operator=>  OutDataTypeStr=boolean  RndMeth=Nearest
  Sum : Sum  Inputs=|++
  Switch : Switch  Criteria=u2 > Threshold
  Switch1 : Switch  Criteria=u2 > Threshold
  Rampe : Outport
  RX Timeout Error : Outport  Port=2
  wires:
  TXStatus/1 -> Switch/2
  Delay/1 -> Sum/2
  Constant/1 -> Sum/1
  Sum/1 -> Switch/3
  Switch/1 -> Delay/1, Relational Operator/1, Rampe/1
  Constant1/1 -> Switch/1
  Constant2/1 -> Switch1/1
  Constant3/1 -> Switch1/3
  Switch1/1 -> RX Timeout Error/1
  Relational Operator/1 -> Switch1/2
  Timeout/1 -> Relational Operator/2

== system DR18E_Testpult/Eingabe Fahrzeug/BMS/STK1-5_Temp /RX Timeout Detection8/Subsystem ==
  TXStatus : Inport
  Timeout : Inport  Port=2
  Constant : Constant
  Constant1 : Constant  Value=0
  Constant2 : Constant
  Constant3 : Constant  Value=0
  Delay : Delay  DelayLength=1  InitialCondition=0
  Relational Operator : RelationalOperator  Operator=>  OutDataTypeStr=boolean  RndMeth=Nearest
  Sum : Sum  Inputs=|++
  Switch : Switch  Criteria=u2 > Threshold
  Switch1 : Switch  Criteria=u2 > Threshold
  Rampe : Outport
  RX Timeout Error : Outport  Port=2
  wires:
  TXStatus/1 -> Switch/2
  Delay/1 -> Sum/2
  Constant/1 -> Sum/1
  Sum/1 -> Switch/3
  Switch/1 -> Delay/1, Relational Operator/1, Rampe/1
  Constant1/1 -> Switch/1
  Constant2/1 -> Switch1/1
  Constant3/1 -> Switch1/3
  Switch1/1 -> RX Timeout Error/1
  Relational Operator/1 -> Switch1/2
  Timeout/1 -> Relational Operator/2

== system DR18E_Testpult/Eingabe Fahrzeug/BMS/STK1-5_Temp /RX Timeout Detection9/Subsystem ==
  TXStatus : Inport
  Timeout : Inport  Port=2
  Constant : Constant
  Constant1 : Constant  Value=0
  Constant2 : Constant
  Constant3 : Constant  Value=0
  Delay : Delay  DelayLength=1  InitialCondition=0
  Relational Operator : RelationalOperator  Operator=>  OutDataTypeStr=boolean  RndMeth=Nearest
  Sum : Sum  Inputs=|++
  Switch : Switch  Criteria=u2 > Threshold
  Switch1 : Switch  Criteria=u2 > Threshold
  Rampe : Outport
  RX Timeout Error : Outport  Port=2
  wires:
  TXStatus/1 -> Switch/2
  Delay/1 -> Sum/2
  Constant/1 -> Sum/1
  Sum/1 -> Switch/3
  Switch/1 -> Delay/1, Relational Operator/1, Rampe/1
  Constant1/1 -> Switch/1
  Constant2/1 -> Switch1/1
  Constant3/1 -> Switch1/3
  Switch1/1 -> RX Timeout Error/1
  Relational Operator/1 -> Switch1/2
  Timeout/1 -> Relational Operator/2

== system DR18E_Testpult/Eingabe Fahrzeug/BMS/STK6-10_Temp/RX Timeout Detection1/Subsystem ==
  TXStatus : Inport
  Timeout : Inport  Port=2
  Constant : Constant
  Constant1 : Constant  Value=0
  Constant2 : Constant
  Constant3 : Constant  Value=0
  Delay : Delay  DelayLength=1  InitialCondition=0
  Relational Operator : RelationalOperator  Operator=>  OutDataTypeStr=boolean  RndMeth=Nearest
  Sum : Sum  Inputs=|++
  Switch : Switch  Criteria=u2 > Threshold
  Switch1 : Switch  Criteria=u2 > Threshold
  Rampe : Outport
  RX Timeout Error : Outport  Port=2
  wires:
  TXStatus/1 -> Switch/2
  Delay/1 -> Sum/2
  Constant/1 -> Sum/1
  Sum/1 -> Switch/3
  Switch/1 -> Delay/1, Relational Operator/1, Rampe/1
  Constant1/1 -> Switch/1
  Constant2/1 -> Switch1/1
  Constant3/1 -> Switch1/3
  Switch1/1 -> RX Timeout Error/1
  Relational Operator/1 -> Switch1/2
  Timeout/1 -> Relational Operator/2

== system DR18E_Testpult/Eingabe Fahrzeug/BMS/STK6-10_Temp/RX Timeout Detection10/Subsystem ==
  TXStatus : Inport
  Timeout : Inport  Port=2
  Constant : Constant
  Constant1 : Constant  Value=0
  Constant2 : Constant
  Constant3 : Constant  Value=0
  Delay : Delay  DelayLength=1  InitialCondition=0
  Relational Operator : RelationalOperator  Operator=>  OutDataTypeStr=boolean  RndMeth=Nearest
  Sum : Sum  Inputs=|++
  Switch : Switch  Criteria=u2 > Threshold
  Switch1 : Switch  Criteria=u2 > Threshold
  Rampe : Outport
  RX Timeout Error : Outport  Port=2
  wires:
  TXStatus/1 -> Switch/2
  Delay/1 -> Sum/2
  Constant/1 -> Sum/1
  Sum/1 -> Switch/3
  Switch/1 -> Delay/1, Relational Operator/1, Rampe/1
  Constant1/1 -> Switch/1
  Constant2/1 -> Switch1/1
  Constant3/1 -> Switch1/3
  Switch1/1 -> RX Timeout Error/1
  Relational Operator/1 -> Switch1/2
  Timeout/1 -> Relational Operator/2

== system DR18E_Testpult/Eingabe Fahrzeug/BMS/STK6-10_Temp/RX Timeout Detection2/Subsystem ==
  TXStatus : Inport
  Timeout : Inport  Port=2
  Constant : Constant
  Constant1 : Constant  Value=0
  Constant2 : Constant
  Constant3 : Constant  Value=0
  Delay : Delay  DelayLength=1  InitialCondition=0
  Relational Operator : RelationalOperator  Operator=>  OutDataTypeStr=boolean  RndMeth=Nearest
  Sum : Sum  Inputs=|++
  Switch : Switch  Criteria=u2 > Threshold
  Switch1 : Switch  Criteria=u2 > Threshold
  Rampe : Outport
  RX Timeout Error : Outport  Port=2
  wires:
  TXStatus/1 -> Switch/2
  Delay/1 -> Sum/2
  Constant/1 -> Sum/1
  Sum/1 -> Switch/3
  Switch/1 -> Delay/1, Relational Operator/1, Rampe/1
  Constant1/1 -> Switch/1
  Constant2/1 -> Switch1/1
  Constant3/1 -> Switch1/3
  Switch1/1 -> RX Timeout Error/1
  Relational Operator/1 -> Switch1/2
  Timeout/1 -> Relational Operator/2

== system DR18E_Testpult/Eingabe Fahrzeug/BMS/STK6-10_Temp/RX Timeout Detection3/Subsystem ==
  TXStatus : Inport
  Timeout : Inport  Port=2
  Constant : Constant
  Constant1 : Constant  Value=0
  Constant2 : Constant
  Constant3 : Constant  Value=0
  Delay : Delay  DelayLength=1  InitialCondition=0
  Relational Operator : RelationalOperator  Operator=>  OutDataTypeStr=boolean  RndMeth=Nearest
  Sum : Sum  Inputs=|++
  Switch : Switch  Criteria=u2 > Threshold
  Switch1 : Switch  Criteria=u2 > Threshold
  Rampe : Outport
  RX Timeout Error : Outport  Port=2
  wires:
  TXStatus/1 -> Switch/2
  Delay/1 -> Sum/2
  Constant/1 -> Sum/1
  Sum/1 -> Switch/3
  Switch/1 -> Delay/1, Relational Operator/1, Rampe/1
  Constant1/1 -> Switch/1
  Constant2/1 -> Switch1/1
  Constant3/1 -> Switch1/3
  Switch1/1 -> RX Timeout Error/1
  Relational Operator/1 -> Switch1/2
  Timeout/1 -> Relational Operator/2

== system DR18E_Testpult/Eingabe Fahrzeug/BMS/STK6-10_Temp/RX Timeout Detection4/Subsystem ==
  TXStatus : Inport
  Timeout : Inport  Port=2
  Constant : Constant
  Constant1 : Constant  Value=0
  Constant2 : Constant
  Constant3 : Constant  Value=0
  Delay : Delay  DelayLength=1  InitialCondition=0
  Relational Operator : RelationalOperator  Operator=>  OutDataTypeStr=boolean  RndMeth=Nearest
  Sum : Sum  Inputs=|++
  Switch : Switch  Criteria=u2 > Threshold
  Switch1 : Switch  Criteria=u2 > Threshold
  Rampe : Outport
  RX Timeout Error : Outport  Port=2
  wires:
  TXStatus/1 -> Switch/2
  Delay/1 -> Sum/2
  Constant/1 -> Sum/1
  Sum/1 -> Switch/3
  Switch/1 -> Delay/1, Relational Operator/1, Rampe/1
  Constant1/1 -> Switch/1
  Constant2/1 -> Switch1/1
  Constant3/1 -> Switch1/3
  Switch1/1 -> RX Timeout Error/1
  Relational Operator/1 -> Switch1/2
  Timeout/1 -> Relational Operator/2

== system DR18E_Testpult/Eingabe Fahrzeug/BMS/STK6-10_Temp/RX Timeout Detection5/Subsystem ==
  TXStatus : Inport
  Timeout : Inport  Port=2
  Constant : Constant
  Constant1 : Constant  Value=0
  Constant2 : Constant
  Constant3 : Constant  Value=0
  Delay : Delay  DelayLength=1  InitialCondition=0
  Relational Operator : RelationalOperator  Operator=>  OutDataTypeStr=boolean  RndMeth=Nearest
  Sum : Sum  Inputs=|++
  Switch : Switch  Criteria=u2 > Threshold
  Switch1 : Switch  Criteria=u2 > Threshold
  Rampe : Outport
  RX Timeout Error : Outport  Port=2
  wires:
  TXStatus/1 -> Switch/2
  Delay/1 -> Sum/2
  Constant/1 -> Sum/1
  Sum/1 -> Switch/3
  Switch/1 -> Delay/1, Relational Operator/1, Rampe/1
  Constant1/1 -> Switch/1
  Constant2/1 -> Switch1/1
  Constant3/1 -> Switch1/3
  Switch1/1 -> RX Timeout Error/1
  Relational Operator/1 -> Switch1/2
  Timeout/1 -> Relational Operator/2

== system DR18E_Testpult/Eingabe Fahrzeug/BMS/STK6-10_Temp/RX Timeout Detection6/Subsystem ==
  TXStatus : Inport
  Timeout : Inport  Port=2
  Constant : Constant
  Constant1 : Constant  Value=0
  Constant2 : Constant
  Constant3 : Constant  Value=0
  Delay : Delay  DelayLength=1  InitialCondition=0
  Relational Operator : RelationalOperator  Operator=>  OutDataTypeStr=boolean  RndMeth=Nearest
  Sum : Sum  Inputs=|++
  Switch : Switch  Criteria=u2 > Threshold
  Switch1 : Switch  Criteria=u2 > Threshold
  Rampe : Outport
  RX Timeout Error : Outport  Port=2
  wires:
  TXStatus/1 -> Switch/2
  Delay/1 -> Sum/2
  Constant/1 -> Sum/1
  Sum/1 -> Switch/3
  Switch/1 -> Delay/1, Relational Operator/1, Rampe/1
  Constant1/1 -> Switch/1
  Constant2/1 -> Switch1/1
  Constant3/1 -> Switch1/3
  Switch1/1 -> RX Timeout Error/1
  Relational Operator/1 -> Switch1/2
  Timeout/1 -> Relational Operator/2

== system DR18E_Testpult/Eingabe Fahrzeug/BMS/STK6-10_Temp/RX Timeout Detection7/Subsystem ==
  TXStatus : Inport
  Timeout : Inport  Port=2
  Constant : Constant
  Constant1 : Constant  Value=0
  Constant2 : Constant
  Constant3 : Constant  Value=0
  Delay : Delay  DelayLength=1  InitialCondition=0
  Relational Operator : RelationalOperator  Operator=>  OutDataTypeStr=boolean  RndMeth=Nearest
  Sum : Sum  Inputs=|++
  Switch : Switch  Criteria=u2 > Threshold
  Switch1 : Switch  Criteria=u2 > Threshold
  Rampe : Outport
  RX Timeout Error : Outport  Port=2
  wires:
  TXStatus/1 -> Switch/2
  Delay/1 -> Sum/2
  Constant/1 -> Sum/1
  Sum/1 -> Switch/3
  Switch/1 -> Delay/1, Relational Operator/1, Rampe/1
  Constant1/1 -> Switch/1
  Constant2/1 -> Switch1/1
  Constant3/1 -> Switch1/3
  Switch1/1 -> RX Timeout Error/1
  Relational Operator/1 -> Switch1/2
  Timeout/1 -> Relational Operator/2

== system DR18E_Testpult/Eingabe Fahrzeug/BMS/STK6-10_Temp/RX Timeout Detection8/Subsystem ==
  TXStatus : Inport
  Timeout : Inport  Port=2
  Constant : Constant
  Constant1 : Constant  Value=0
  Constant2 : Constant
  Constant3 : Constant  Value=0
  Delay : Delay  DelayLength=1  InitialCondition=0
  Relational Operator : RelationalOperator  Operator=>  OutDataTypeStr=boolean  RndMeth=Nearest
  Sum : Sum  Inputs=|++
  Switch : Switch  Criteria=u2 > Threshold
  Switch1 : Switch  Criteria=u2 > Threshold
  Rampe : Outport
  RX Timeout Error : Outport  Port=2
  wires:
  TXStatus/1 -> Switch/2
  Delay/1 -> Sum/2
  Constant/1 -> Sum/1
  Sum/1 -> Switch/3
  Switch/1 -> Delay/1, Relational Operator/1, Rampe/1
  Constant1/1 -> Switch/1
  Constant2/1 -> Switch1/1
  Constant3/1 -> Switch1/3
  Switch1/1 -> RX Timeout Error/1
  Relational Operator/1 -> Switch1/2
  Timeout/1 -> Relational Operator/2

== system DR18E_Testpult/Eingabe Fahrzeug/BMS/STK6-10_Temp/RX Timeout Detection9/Subsystem ==
  TXStatus : Inport
  Timeout : Inport  Port=2
  Constant : Constant
  Constant1 : Constant  Value=0
  Constant2 : Constant
  Constant3 : Constant  Value=0
  Delay : Delay  DelayLength=1  InitialCondition=0
  Relational Operator : RelationalOperator  Operator=>  OutDataTypeStr=boolean  RndMeth=Nearest
  Sum : Sum  Inputs=|++
  Switch : Switch  Criteria=u2 > Threshold
  Switch1 : Switch  Criteria=u2 > Threshold
  Rampe : Outport
  RX Timeout Error : Outport  Port=2
  wires:
  TXStatus/1 -> Switch/2
  Delay/1 -> Sum/2
  Constant/1 -> Sum/1
  Sum/1 -> Switch/3
  Switch/1 -> Delay/1, Relational Operator/1, Rampe/1
  Constant1/1 -> Switch/1
  Constant2/1 -> Switch1/1
  Constant3/1 -> Switch1/3
  Switch1/1 -> RX Timeout Error/1
  Relational Operator/1 -> Switch1/2
  Timeout/1 -> Relational Operator/2

== system DR18E_Testpult/Eingabe Fahrzeug/BMS/Voltage 9-10/Voltage Stack 10/RX Timeout Detection ==
  RX status : Inport
  Timeout (n Samples) : Inport  Port=2
  Subsystem : Subsystem  TreatAsAtomicUnit=on
  Terminator_4 : Terminator
  RX Timeout Error : Outport
  wires:
  RX status/1 -> Subsystem/1(TXStatus)
  Subsystem/1(Rampe) -> Terminator_4/1
  Subsystem/2(RX Timeout Error) -> RX Timeout Error/1  "RX Timeout"
  Timeout (n Samples)/1 -> Subsystem/2(Timeout)

== system DR18E_Testpult/Eingabe Fahrzeug/BMS/Voltage 9-10/Voltage Stack 10/RX Timeout Detection1 ==
  RX status : Inport
  Timeout (n Samples) : Inport  Port=2
  Subsystem : Subsystem  TreatAsAtomicUnit=on
  Terminator_4 : Terminator
  RX Timeout Error : Outport
  wires:
  RX status/1 -> Subsystem/1(TXStatus)
  Subsystem/1(Rampe) -> Terminator_4/1
  Subsystem/2(RX Timeout Error) -> RX Timeout Error/1  "RX Timeout"
  Timeout (n Samples)/1 -> Subsystem/2(Timeout)

== system DR18E_Testpult/Eingabe Fahrzeug/BMS/Voltage 9-10/Voltage Stack 10/RX Timeout Detection2 ==
  RX status : Inport
  Timeout (n Samples) : Inport  Port=2
  Subsystem : Subsystem  TreatAsAtomicUnit=on
  Terminator_4 : Terminator
  RX Timeout Error : Outport
  wires:
  RX status/1 -> Subsystem/1(TXStatus)
  Subsystem/1(Rampe) -> Terminator_4/1
  Subsystem/2(RX Timeout Error) -> RX Timeout Error/1  "RX Timeout"
  Timeout (n Samples)/1 -> Subsystem/2(Timeout)

== system DR18E_Testpult/Eingabe Fahrzeug/BMS/Voltage 9-10/Voltage Stack 9/RX Timeout Detection ==
  RX status : Inport
  Timeout (n Samples) : Inport  Port=2
  Subsystem : Subsystem  TreatAsAtomicUnit=on
  Terminator_4 : Terminator
  RX Timeout Error : Outport
  wires:
  RX status/1 -> Subsystem/1(TXStatus)
  Subsystem/1(Rampe) -> Terminator_4/1
  Subsystem/2(RX Timeout Error) -> RX Timeout Error/1  "RX Timeout"
  Timeout (n Samples)/1 -> Subsystem/2(Timeout)

== system DR18E_Testpult/Eingabe Fahrzeug/BMS/Voltage 9-10/Voltage Stack 9/RX Timeout Detection1 ==
  RX status : Inport
  Timeout (n Samples) : Inport  Port=2
  Subsystem : Subsystem  TreatAsAtomicUnit=on
  Terminator_4 : Terminator
  RX Timeout Error : Outport
  wires:
  RX status/1 -> Subsystem/1(TXStatus)
  Subsystem/1(Rampe) -> Terminator_4/1
  Subsystem/2(RX Timeout Error) -> RX Timeout Error/1  "RX Timeout"
  Timeout (n Samples)/1 -> Subsystem/2(Timeout)

== system DR18E_Testpult/Eingabe Fahrzeug/BMS/Voltage 9-10/Voltage Stack 9/RX Timeout Detection2 ==
  RX status : Inport
  Timeout (n Samples) : Inport  Port=2
  Subsystem : Subsystem  TreatAsAtomicUnit=on
  Terminator_4 : Terminator
  RX Timeout Error : Outport
  wires:
  RX status/1 -> Subsystem/1(TXStatus)
  Subsystem/1(Rampe) -> Terminator_4/1
  Subsystem/2(RX Timeout Error) -> RX Timeout Error/1  "RX Timeout"
  Timeout (n Samples)/1 -> Subsystem/2(Timeout)

== system DR18E_Testpult/Eingabe Fahrzeug/BMS/Voltage Stack 1-2/Voltage Stack 1/RX Timeout Detection ==
  RX status : Inport
  Timeout (n Samples) : Inport  Port=2
  Subsystem : Subsystem  TreatAsAtomicUnit=on
  Terminator_4 : Terminator
  RX Timeout Error : Outport
  wires:
  RX status/1 -> Subsystem/1(TXStatus)
  Subsystem/1(Rampe) -> Terminator_4/1
  Subsystem/2(RX Timeout Error) -> RX Timeout Error/1  "RX Timeout"
  Timeout (n Samples)/1 -> Subsystem/2(Timeout)

== system DR18E_Testpult/Eingabe Fahrzeug/BMS/Voltage Stack 1-2/Voltage Stack 1/RX Timeout Detection1 ==
  RX status : Inport
  Timeout (n Samples) : Inport  Port=2
  Subsystem : Subsystem  TreatAsAtomicUnit=on
  Terminator_4 : Terminator
  RX Timeout Error : Outport
  wires:
  RX status/1 -> Subsystem/1(TXStatus)
  Subsystem/1(Rampe) -> Terminator_4/1
  Subsystem/2(RX Timeout Error) -> RX Timeout Error/1  "RX Timeout"
  Timeout (n Samples)/1 -> Subsystem/2(Timeout)
